simulink model "OFDM_Tx_Rx_HW"  (R2020a)
settings: Solver=FixedStepDiscrete  StartTime=0.0  StopTime=inf  RelTol=1e-3
PostLoadFcn:
  | run ./scripts/filter_setup;
InitFcn:
  | % Set parameters
  | fs = 1e6;
  | 
  | % Load all required variables
  | load('variables/read_addr_data');
  | load('variables/read_addr_cp');
  | load('variables/read_addr_pream');
  | load('variables/read_addr_rx');
  | load('variables/pilot');
  | load('variables/sc_index');
  | load('variables/LTSfreq');
  | load('variables/STSfreq');
  | load('variables/LTSread');
  | load('variables/STSread');
libraries: xbsIndex_r4 x1, decimate_rx x1, interpolate_tx x1, OFDM_Rx x1, OFDM_Tx x1
settings Model: SimulationMode=accelerator  Creator=njb13206  LastModifiedBy=LDM
settings OptimizationCC: BlockReduction=off  ConditionallyExecuteInputs=off  DefaultParameterBehavior=Inlined
settings DebuggingCC: AlgebraicLoopMsg=error  IntegerOverflowMsg=none  ParameterPrecisionLossMsg=none  IntegerSaturationMsg=none
settings HardwareCC: ProdBitPerPointer=32  ProdBitPerSizeT=32  ProdBitPerPtrDiffT=32  ProdLargestAtomicFloat=None  ProdIntDivRoundTo=Undefined  ProdEndianess=Unspecified  ProdWordSize=32  ProdHWDeviceType=ASIC/FPGA->ASIC/FPGA  TargetBitPerPointer=64  TargetBitPerSizeT=64  TargetBitPerPtrDiffT=64  TargetLongLongMode=on  TargetIntDivRoundTo=Zero  TargetEndianess=LittleEndian  TargetWordSize=64  TargetHWDeviceType=Custom Processor->MATLAB Host Computer  ProdEqTarget=off

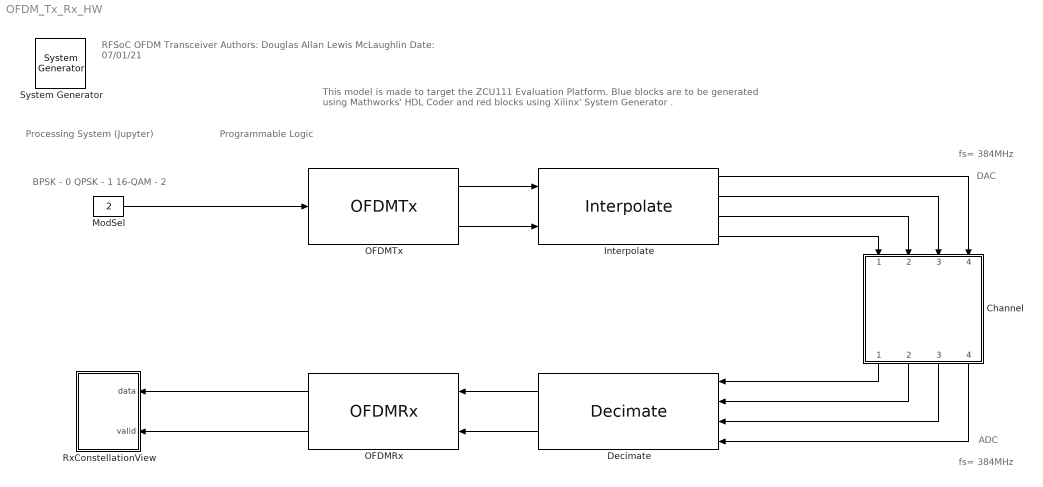
== system OFDM_Tx_Rx_HW ==
  note: This model is made to target the ZCU111 Evaluation Platform. Blue blocks are to be generated using Mathworks' HDL Coder and red blocks using Xilinx' System Generator .
  note: Programmable Logic
  note: Processing System (Jupyter)
  note: DAC
  note: BPSK - 0
      | QPSK - 1
      | 16-QAM - 2
  note: fs= 384MHz
  note: ADC
  note: fs= 384MHz
  note: RFSoC OFDM Transceiver
      | Authors: Douglas Allan
      | Lewis McLaughlin
      | Date: 07/01/21
  " System Generator" : xbsIndex_r4/ System Generator  Tag=genX  xilinxfamily=zynquplusRFSOC  part=xczu28dr  speed=-2-e  package=ffvg1517  synthesis_tool=Vivado  clock_wrapper=Clock Enables  directory=./netlist  proj_type=Vivado  Synth_file=Vivado Synthesis Defaults  Impl_file=Vivado Implementation Defaults  testbench=off  simulink_period=1/192e6  sysclk_period=1000/192  dcm_input_clock_period=10  incr_netlist=off  trim_vbits=Everywhere in SubSystem  dbl_ovrd=According to Block Masks  core_generation=According to Block Masks  run_coregen=off  deprecated_control=off  eval_field=0  block_type=sysgen
  "Channel " : Subsystem
  Decimate : decimate_rx/Decimate  SystemSampleTime=-1  Latency=0  AutoFrameSizeCalculation=off
  Interpolate : interpolate_tx/Interpolate  SystemSampleTime=-1  Latency=0  AutoFrameSizeCalculation=off
  ModSel : Constant  Value=2  OutDataTypeStr=fixdt(0,2,0)  SampleTime=1/fs
  OFDMRx : OFDM_Rx/OFDMRx  SystemSampleTime=-1  Latency=0  AutoFrameSizeCalculation=off
  OFDMTx : OFDM_Tx/OFDMTx  SystemSampleTime=-1  Latency=0  AutoFrameSizeCalculation=off
  RxConstellationView : Subsystem
  wires:
  OFDMRx/1 -> RxConstellationView/1(data)
  OFDMRx/2 -> RxConstellationView/2(valid)
  ModSel/1 -> OFDMTx/1
  Interpolate/1 -> "Channel "/4(chanIn_re)
  OFDMTx/1 -> Interpolate/1
  OFDMTx/2 -> Interpolate/2
  Interpolate/3 -> "Channel "/2(chanIn_im)
  Interpolate/2 -> "Channel "/3(m_re_tvalid)
  Interpolate/4 -> "Channel "/1(m_im_tvalid)
  "Channel "/1(chanOut_re) -> Decimate/1
  "Channel "/3(chanOut_im) -> Decimate/3
  "Channel "/4(tvalid_im_out) -> Decimate/4
  "Channel "/2(tvalid_re_out) -> Decimate/2
  Decimate/1 -> OFDMRx/1
  Decimate/2 -> OFDMRx/2

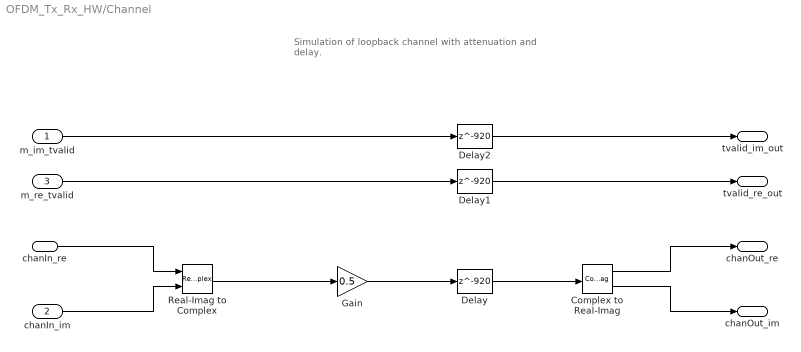
== system OFDM_Tx_Rx_HW/Channel  ==
  note: Simulation of loopback channel with attenuation and
      | delay.
  m_im_tvalid : Inport
  chanIn_im : Inport  Port=2
  m_re_tvalid : Inport  Port=3
  chanIn_re : Inport  Port=4
  Complex to Real-Imag : ComplexToRealImag
  Delay : Delay  DelayLength=920
  Delay1 : Delay  DelayLength=920
  Delay2 : Delay  DelayLength=920
  Gain : Gain  Gain=0.5  ParamDataTypeStr=double  OutDataTypeStr=fixdt(1,16,14)
  Real-Imag to Complex : RealImagToComplex
  chanOut_re : Outport  VectorParamsAs1DForOutWhenUnconnected=off
  tvalid_re_out : Outport  Port=2  VectorParamsAs1DForOutWhenUnconnected=off
  chanOut_im : Outport  Port=3  VectorParamsAs1DForOutWhenUnconnected=off
  tvalid_im_out : Outport  Port=4  VectorParamsAs1DForOutWhenUnconnected=off
  wires:
  Gain/1 -> Delay/1
  Real-Imag to Complex/1 -> Gain/1
  chanIn_re/1 -> Real-Imag to Complex/1
  chanIn_im/1 -> Real-Imag to Complex/2
  m_re_tvalid/1 -> Delay1/1
  m_im_tvalid/1 -> Delay2/1
  Delay/1 -> Complex to Real-Imag/1
  Complex to Real-Imag/1 -> chanOut_re/1
  Complex to Real-Imag/2 -> chanOut_im/1
  Delay2/1 -> tvalid_im_out/1
  Delay1/1 -> tvalid_re_out/1

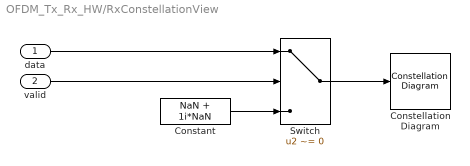
== system OFDM_Tx_Rx_HW/RxConstellationView ==
  data : Inport
  valid : Inport  Port=2
  Constant : Constant  Value=NaN + 1i*NaN  OutDataTypeStr=double  SampleTime=-1
  Constellation Diagram : ConstellationDiagram
  Switch : Switch  Criteria=u2 ~= 0
  wires:
  Switch/1 -> Constellation Diagram/1
  Constant/1 -> Switch/3
  valid/1 -> Switch/2
  data/1 -> Switch/1
